simulink model "m01_pid_adrc_sine"  (R2023b)
settings: Solver=ode45  StartTime=0.0  StopTime=4  MaxStep=5e-4  RelTol=1e-3
libraries: slpidlib x1
settings Model: Creator=30504  LastModifiedBy=30504
settings DataIOCC: ReturnWorkspaceOutputs=off

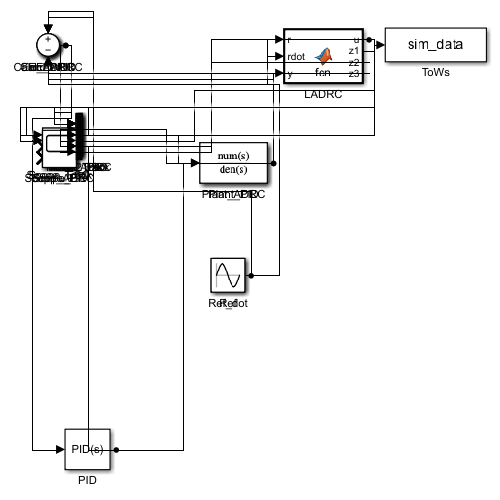
[thumbnail: Simulink's stored preview of the top-level diagram]
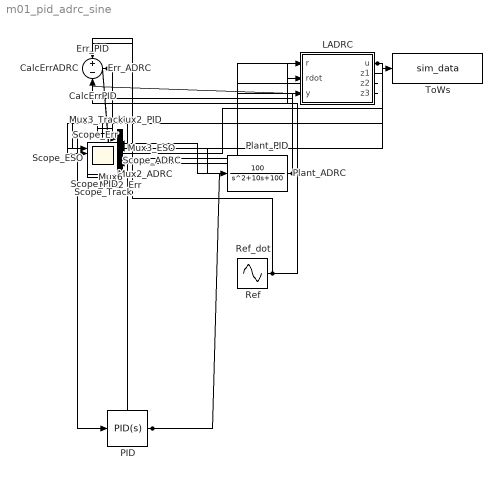
== system m01_pid_adrc_sine ==
  CalcErrADRC : Sum  Inputs=+-
  CalcErrPID : Sum  Inputs=+-
  Err_ADRC : Sum  Inputs=+-
  Err_PID : Sum  Inputs=+-
  LADRC : MATLAB Function  TreatAsAtomicUnit=on
  Mux2_ADRC : Mux  Inputs=2
  Mux2_Err : Mux  Inputs=2
  Mux2_PID : Mux  Inputs=2
  Mux3_ESO : Mux  Inputs=3
  Mux3_Track : Mux  Inputs=3
  Mux6 : Mux  Inputs=6
  PID : slpidlib/PID Controller  Controller=PID  Form=Parallel  TimeDomain=Continuous-time  UseExternalTs=off  SampleTime=0.001  IntegratorMethod=Forward Euler  FilterMethod=Forward Euler  ControllerParametersSource=internal  P=300  I=1500  UseKiTs=off  D=15  N=500  UseFilter=on  TunerSelectOption=Transfer Function Based (PID Tuner App)  InitialConditionSource=internal  InitialConditionForIntegrator=0  InitialConditionForFilter=0  DifferentiatorICPrevScaledInput=0  ExternalReset=none  TrackingMode=off  Kt=1  LimitOutput=off  SatLimitsSource=internal  UpperSaturationLimit=inf  LowerSaturationLimit=-inf  LinearizeAsGain=off  AntiWindupMode=none  Kb=1  LimitIntegrator=off  UpperIntegratorSaturationLimit=inf  LowerIntegratorSaturationLimit=-inf  POutMin=[]  POutMax=[]  IOutMin=[]  IOutMax=[]  DOutMin=[]  DOutMax=[]  NOutMin=[]  NOutMax=[]  SumOutMin=[]  SumOutMax=[]  SaturationOutMin=[]  SaturationOutMax=[]  PParamMin=[]  PParamMax=[]  IParamMin=[]  IParamMax=[]  DParamMin=[]  DParamMax=[]  NParamMin=[]  NParamMax=[]  KbParamMin=[]  KbParamMax=[]  KtParamMin=[]  KtParamMax=[]  KbOutMin=[]  KbOutMax=[]  KtOutMin=[]  KtOutMax=[]  IntegratorOutMin=[]  IntegratorOutMax=[]  FilterOutMin=[]  FilterOutMax=[]  SumI1OutMin=[]  SumI1OutMax=[]  SumI2OutMin=[]  SumI2OutMax=[]  SumI3OutMin=[]  SumI3OutMax=[]  SumI4OutMin=[]  SumI4OutMax=[]  SumDOutMin=[]  SumDOutMax=[]  DifferentiatorOutMin=[]  DifferentiatorOutMax=[]  FilterDiffOutCoefMin=[]  FilterDiffOutCoefMax=[]  ReciprocalOutMin=[]  ReciprocalOutMax=[]  SumDenOutMin=[]  SumDenOutMax=[]  SumNumOutMin=[]  SumNumOutMax=[]  DivideOutMin=[]  DivideOutMax=[]  UdiffTsProdOutMin=[]  UdiffTsProdOutMax=[]  NTsProdOutMin=[]  NTsProdOutMax=[]  UintegralTsProdOutMin=[]  UintegralTsProdOutMax=[]  UngainTsProdOutMin=[]  UngainTsProdOutMax=[]  ClampingZeroOutDataTypeStr=Inherit: Inherit via back propagation  ClampingZeroOutMin=[]  ClampingZeroOutMax=[]  FilterDenConstantOutDataTypeStr=Inherit: Inherit via back propagation  FilterDenConstantOutMin=[]  FilterDenConstantOutMax=[]  PCopyOutDataTypeStr=Inherit: Inherit via back propagation  PCopyOutMin=[]  PCopyOutMax=[]  NCopyOutDataTypeStr=Inherit: Inherit via back propagation  NCopyOutMin=[]  NCopyOutMax=[]  IntegratorContinuousStateAttributes=''  IntegratorStateMustResolveToSignalObject=off  IntegratorRTWStateStorageClass=Auto  FilterContinuousStateAttributes=''  FilterStateMustResolveToSignalObject=off  FilterRTWStateStorageClass=Auto  ParallelPVariant=InternalParameters  IdealPVariant=Disabled  IVariant=InternalParameters  DVariant=InternalParameters  IntegratorVariant=Continuous  SatVariant=Disabled  AWVariant=Passthrough  PCopyVariant=Disabled  TRVariant=Disabled  FdbkBlocksVariant=Forward  IdealPFdbkVariant=Disabled  SatFdbkVariant=Disabled  DerivativeFilterVariant=ContFilter  NVariant=InternalParameters  NCopyVariant=Disabled  FilterICVariant=InternalICsFilter  IntegratorICVariant=InternalICs  ExternalResetVariant=Disabled  TRSumVariant=Passthrough  SumFdbkVariant=Disabled  SumVariant=Sum_PID  TsampFilterVariant=InternalTs  TsampNgainVariant=Passthrough  TsampIntegralVariant=Disabled_SignalSpec  ExternalSaturationOutDataTypeStr=Inherit: Same as second input
      settings: LibrarySourceBlock=simulink/Discrete/Discrete PID Controller
  Plant_ADRC : TransferFcn  Numerator=[100]  Denominator=[1 10 100]
  Plant_PID : TransferFcn  Numerator=[100]  Denominator=[1 10 100]
  Ref : Sin  Frequency=2*pi*0.5  SampleTime=0
  Ref_dot : Sin  Amplitude=2*pi*0.5  Frequency=2*pi*0.5  Phase=pi/2  SampleTime=0
  Scope_ADRC : Scope  NumInputPorts=2
  Scope_ESO : Scope  NumInputPorts=3
  Scope_Err : Scope  NumInputPorts=2
  Scope_PID : Scope  NumInputPorts=2
  Scope_Track : Scope  NumInputPorts=3
  ToWs : ToWorkspace  VariableName=sim_data  SaveFormat=Structure With Time  SampleTime=-1
  wires:
  Ref/1 -> Err_PID/1, CalcErrPID/1, LADRC/1(r), Err_ADRC/1, CalcErrADRC/1, Mux3_Track/1, Mux6/1
  Err_PID/1 -> PID/1, Mux2_PID/1
  PID/1 -> Plant_PID/1, Mux2_PID/2
  Plant_PID/1 -> Err_PID/2, CalcErrPID/2, Mux3_Track/2, Mux6/2
  Ref_dot/1 -> LADRC/2(rdot)
  Plant_ADRC/1 -> LADRC/3(y), Err_ADRC/2, CalcErrADRC/2, Mux3_Track/3, Mux6/3
  LADRC/1(u) -> Plant_ADRC/1, Mux2_ADRC/2, Mux6/6
  Mux3_Track/1 -> Scope_Track/1
  Mux2_PID/1 -> Scope_PID/1
  Err_ADRC/1 -> Mux2_ADRC/1
  Mux2_ADRC/1 -> Scope_ADRC/1
  LADRC/2(z1) -> Mux3_ESO/1
  LADRC/3(z2) -> Mux3_ESO/2
  LADRC/4(z3) -> Mux3_ESO/3
  Mux3_ESO/1 -> Scope_ESO/1
  CalcErrPID/1 -> Mux2_Err/1, Mux6/4
  CalcErrADRC/1 -> Mux2_Err/2, Mux6/5
  Mux2_Err/1 -> Scope_Err/1
  Mux6/1 -> ToWs/1

== matlab function m01_pid_adrc_sine/LADRC ==
  settings: updateMethod=DISCRETE  sampleTime=0.001
  data: r input; u output; rdot input; y input; z1 output; z2 output; z3 output
% LADRC: 二阶对象, 三阶 LESO, 线性状态误差反馈 + 参考导数前馈
% 输入: r (参考), rdot (参考导数), y (测量)
% 输出: u (控制), z1 (y跟踪), z2 (y导数), z3 (扰动估计)
function [u, z1, z2, z3] = fcn(r, rdot, y)
%#codegen
persistent z1s z2s z3s u_prev
if isempty(z1s)
    z1s = 0; z2s = 0; z3s = 0; u_prev = 0;
end
h = 0.0010000000;
b0 = 100.0000000000;
beta1 = 150.0000000000; beta2 = 7500.0000000000; beta3 = 125000.0000000000;
k1 = 900.0000000000; k2 = 60.0000000000;
% 三阶 LESO 离散更新 (前向 Euler)
e = y - z1s;
z1s = z1s + h * (z2s + beta1 * e);
z2s = z2s + h * (z3s + beta2 * e + b0 * u_prev);
z3s = z3s + h * (beta3 * e);
% 线性状态误差反馈 (含参考导数前馈) + 扰动前馈
u0 = k1 * (r - z1s) + k2 * (rdot - z2s);
u = (u0 - z3s) / b0;
u = max(min(u, 500), -500);  % 输入饱和 +-500
u_prev = u;
% 输出状态
z1 = z1s; z2 = z2s; z3 = z3s;
end
